simulink model "mcb_microchip_pmsm_parameter_est_SAME70"  (R2023b)
settings: Solver=FixedStepDiscrete  StartTime=0.0  StopTime=15  RelTol=1e-3  EnableMultiTasking=on
InitFcn:
  | mcb_microchip_pmsm_parameter_est_SAME70_data;
values from neighbouring files (symbols this model uses):
  Ts = T_pwm    (= 5e-05)    [mcb_microchip_pmsm_parameter_est_SAME70_data.m]
  Ts_motor = T_pwm/2    (= 2.5e-05)    [mcb_microchip_pmsm_parameter_est_SAME70_data.m]
undefined symbols (not defined in the file or in its folder): A24, AD10, AD7, ADC0, inverter, LQFP144, MaxPer, ms, ns, PA0, PA1, PA10, PA11, PA12, PA13, PA16, PA18, PA9, PB0, PD18, PD19, PD24, PD25, PD26, PI_params, Pin, pmsm, Resol, SAME70Q21B, target, Unsigned
libraries: simulink x18, MCHP_Blockset x13, mcbpmsmparamestlib x5, svdutilitieslib x4, mcbpositiondecoderlib x3, mcbplantlib x1, autolibpmsmexterior x1, mcbcontrolslib x1
(part 1 of 4)
settings Model: Creator=Lubin Kerhuel  LastModifiedBy=I69995
settings SolverCC: AlgebraicLoopSolver=TrustRegion
settings DataIOCC: SaveFormat=StructureWithTime  ReturnWorkspaceOutputs=off
settings OptimizationCC: DefaultParameterBehavior=Inlined  DefaultUnderspecifiedDataType=single  EnhancedBackFolding=on  PassReuseOutputArgsAs=Individual arguments  OptimizeBlockOrder=speed  DifferentSizesBufferReuse=on  OptimizationCustomize=off  EfficientTunableParamExpr=on
settings DebuggingCC: MultiTaskDSMMsg=none  ParameterPrecisionLossMsg=none  ParameterTunabilityLossMsg=error  FcnCallInpInsideContextMsg=warning  UnconnectedInputMsg=warning  UnconnectedOutputMsg=warning  UnconnectedLineMsg=warning  SFExecutionAtInitializationDiag=none  ArithmeticOperatorsInVariantConditions=warning
settings HardwareCC: ProdBitPerPointer=32  ProdBitPerSizeT=32  ProdBitPerPtrDiffT=32  ProdLargestAtomicInteger=Integer  ProdWordSize=32  ProdLongLongMode=on  ProdHWDeviceType=ARM Compatible->ARM Cortex
settings ModelReferenceCC: EnableRefExpFcnMdlSchedulingChecks=on  ModelReferenceNumInstancesAllowed=Single  PropagateSignalLabelsOutOfModel=off
settings SFSimCC: SimUseLocalCustomCode=off  MATLABDynamicMemAlloc=off  CustomCodeUndefinedFunction=UseInterfaceOnly
settings RTWCC: Description=Microchip Embedded Target Cortex M7 (real-time)  SystemTargetFile=MCHP_ARM7_stf.tlc  TemplateMakefile=MCHP_ARM7.tmf  GenerateReport=on  RTWUseLocalCustomCode=off  Toolchain=xc32 - v4.30 for Mirochip SAMx7 device  BuildConfiguration=Specify  IncludeHyperlinkInReport=on  LaunchReport=on  GenerateTraceInfo=on  GenerateTraceReport=on  GenerateTraceReportSl=on  GenerateTraceReportSf=on  GenerateTraceReportEml=on  DLArmComputeVersion=19.05
settings CodeAppCC: ForceParamTrailComments=on  IgnoreCustomStorageClasses=off  MaxIdLength=255  OperatorAnnotations=on  SimulinkDataObjDesc=on  SFDataObjDesc=on  InsertBlockDesc=on  InternalIdentifier=Classic
settings STFCustomTargetCC: TargetLangStandard=C89/C90 (ANSI)  MultiwordLength=256  IncludeMdlTerminateFcn=off  CombineOutputUpdateFcns=on  CombineSignalStateStructs=on  SuppressErrorStatus=on  ERTCustomFileBanners=on  SupportContinuousTime=off  RemoveResetFunc=on  MATLABClassNameForMDSCustomization=Simulink.SoftwareTarget.ERTCustomization  UseToolchainInfoCompliant=on  SystemTargetFile=MCHP_ARM7_stf.tlc
settings ERTTargetCC: ParMdlRefBuildCompliant=off  CompOptLevelCompliant=off  ConcurrentExecutionCompliant=off  IncludeMdlTerminateFcn=off  CombineSignalStateStructs=on  SuppressErrorStatus=on  SupportNonInlinedSFcns=on  ModelStepFunctionPrototypeControlCompliant=off  CPPClassGenCompliant=off  ExtModeStaticAllocSize=2000  InlinedParameterPlacement=NonHierarchical  ERTSrcFileBannerTemplate=MCHP_dsPIC_code_template.cgt  ERTHdrFileBannerTemplate=MCHP_dsPIC_code_template.cgt  ERTDataSrcFileTemplate=MCHP_dsPIC_code_template.cgt  ERTDataHdrFileTemplate=MCHP_dsPIC_code_template.cgt  ERTCustomFileTemplate=MCHP_main.tlc

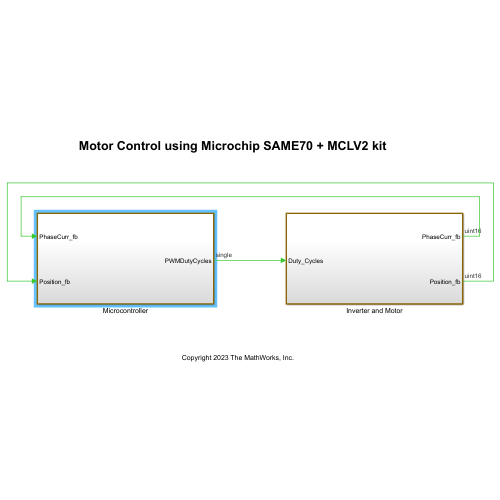
[thumbnail: Simulink's stored preview of the top-level diagram]
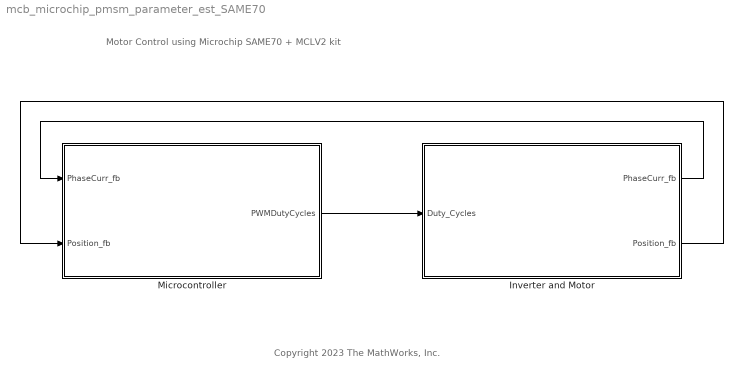
== system mcb_microchip_pmsm_parameter_est_SAME70 ==
  note: Copyright 2023 The MathWorks, Inc.
  note: Motor Control using Microchip SAME70 + MCLV2 kit
  Inverter and Motor : Subsystem
  Microcontroller : Subsystem
  wires:
  Microcontroller/1(PWMDutyCycles) -> Inverter and Motor/1(Duty_Cycles)
  Inverter and Motor/1(PhaseCurr_fb) -> Microcontroller/1(PhaseCurr_fb)
  Inverter and Motor/2(Position_fb) -> Microcontroller/2(Position_fb)

== system mcb_microchip_pmsm_parameter_est_SAME70/Inverter and Motor ==
  Duty_Cycles : Inport
  Inverter and Motor : Subsystem  Variant=on  VariantControlMode=sim codegen switching
  PhaseCurr_fb : Outport
  Position_fb : Outport  Port=2
  wires:
  Duty_Cycles/1 -> Inverter and Motor/1(Duty_Cycles)
  Inverter and Motor/1(PhaseCurr_fb) -> PhaseCurr_fb/1
  Inverter and Motor/2(Position_fb) -> Position_fb/1

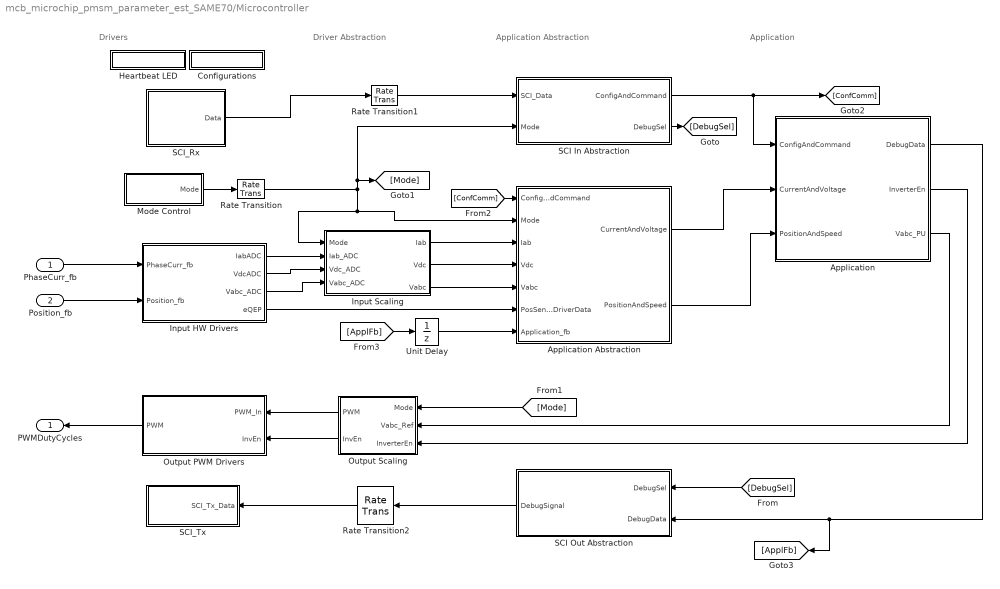
== system mcb_microchip_pmsm_parameter_est_SAME70/Microcontroller ==
  note: Drivers
  note: Driver Abstraction
  note: Application Abstraction
  note: Application
  PhaseCurr_fb : Inport
  Position_fb : Inport  Port=2
  Application : Subsystem
  Application Abstraction : Subsystem
  Configurations : Subsystem
  Heartbeat LED : Subsystem  Variant=on  VariantControlMode=sim codegen switching
  Input HW Drivers : Subsystem  Variant=on  VariantControlMode=sim codegen switching
  Input Scaling : Subsystem
  Mode Control : Subsystem  Variant=on
  Output PWM Drivers : Subsystem  Variant=on  VariantControlMode=sim codegen switching
  Output Scaling : Subsystem
  Rate Transition : RateTransition  Deterministic=off  OutPortSampleTime=Ts
  Rate Transition1 : RateTransition  Deterministic=off  OutPortSampleTime=Ts
  Rate Transition2 : RateTransition  Deterministic=off  OutPortSampleTime=Ts_SerialCom
  SCI In Abstraction : Subsystem
  SCI Out Abstraction : Subsystem
  SCI_Rx : Subsystem
  SCI_Tx : Subsystem  Variant=on  VariantControlMode=sim codegen switching
  Unit Delay : UnitDelay  SampleTime=-1  HasFrameUpgradeWarning=on
  PWMDutyCycles : Outport
  wires:
  SCI In Abstraction/1(ConfigAndCommand) -> Application/1(ConfigAndCommand), [ConfComm]
  Application Abstraction/1(CurrentAndVoltage) -> Application/2(CurrentAndVoltage)
  Application Abstraction/2(PositionAndSpeed) -> Application/3(PositionAndSpeed)
  Input Scaling/1(Iab) -> Application Abstraction/3(Iab)
  Input Scaling/2(Vdc) -> Application Abstraction/4(Vdc)
  Input Scaling/3(Vabc) -> Application Abstraction/5(Vabc)
  Application/1(DebugData) -> SCI Out Abstraction/2(DebugData), [ApplFb]
  Unit Delay/1 -> Application Abstraction/7(Application_fb)
  Rate Transition/1 -> Application Abstraction/2(Mode), Input Scaling/1(Mode), [Mode], SCI In Abstraction/2(Mode)
  Rate Transition1/1 -> SCI In Abstraction/1(SCI_Data)
  SCI_Rx/1(Data) -> Rate Transition1/1
  Position_fb/1 -> Input HW Drivers/2(Position_fb)
  PhaseCurr_fb/1 -> Input HW Drivers/1(PhaseCurr_fb)
  Input HW Drivers/1(IabADC) -> Input Scaling/2(Iab_ADC)
  Input HW Drivers/2(VdcADC) -> Input Scaling/3(Vdc_ADC)
  Input HW Drivers/3(Vabc_ADC) -> Input Scaling/4(Vabc_ADC)
  Input HW Drivers/4(eQEP) -> Application Abstraction/6(PosSenseDriverData)
  Application/3(Vabc_PU) -> Output Scaling/2(Vabc_Ref)
  Application/2(InverterEn) -> Output Scaling/3(InverterEn)
  SCI In Abstraction/2(DebugSel) -> [DebugSel]
  [DebugSel] -> SCI Out Abstraction/1(DebugSel)
  [Mode] -> Output Scaling/1(Mode)
  [ConfComm] -> Application Abstraction/1(ConfigAndCommand)
  [ApplFb] -> Unit Delay/1
  Output PWM Drivers/1(PWM) -> PWMDutyCycles/1
  Output Scaling/1(PWM) -> Output PWM Drivers/1(PWM_In)
  Output Scaling/2(InvEn) -> Output PWM Drivers/2(InvEn)
  SCI Out Abstraction/1(DebugSignal) -> Rate Transition2/1
  Mode Control/1(Mode) -> Rate Transition/1
  Rate Transition2/1 -> SCI_Tx/1(SCI_Tx_Data)

== system mcb_microchip_pmsm_parameter_est_SAME70/Inverter and Motor/Inverter and Motor ==
  Duty_Cycles : Inport
  Codegen : Subsystem  VariantControl=(codegen)
  Sim : Subsystem  VariantControl=(sim)
  PhaseCurr_fb : Outport
  Position_fb : Outport  Port=2

== system mcb_microchip_pmsm_parameter_est_SAME70/Microcontroller/Application ==
  ConfigAndCommand : Inport
  CurrentAndVoltage : Inport  Port=2
  PositionAndSpeed : Inport  Port=3
  Bus Creator : BusCreator  Inputs=5
  Bus Selector2 : BusSelector  OutputSignals=Enable,TestMethod,TestSelect,Config
  Bus Selector4 : BusSelector  OutputSignals=Theta,Speed,EnClosedLoop
  Bus Selector5 : BusSelector  OutputSignals=Iabc,Vdc
  Param Est : Subsystem
  DebugData : Outport
  InverterEn : Outport  Port=2
  Vabc_PU : Outport  Port=3
  wires:
  ConfigAndCommand/1 -> Bus Selector2/1
  PositionAndSpeed/1 -> Bus Selector4/1
  CurrentAndVoltage/1 -> Bus Selector5/1
  Bus Creator/1 -> Param Est/1(HWInputs)
  Bus Selector5/2 -> Bus Creator/2  "<Vdc>"
  Bus Selector5/1 -> Bus Creator/1  "<Iabc>"
  Bus Selector4/1 -> Bus Creator/3  "<Theta>"
  Bus Selector4/2 -> Bus Creator/4  "<Speed>"
  Bus Selector4/3 -> Bus Creator/5  "<EnClosedLoop>"
  Bus Selector2/4 -> Param Est/5(Config)  "<Config>"
  Bus Selector2/3 -> Param Est/4(TestSelect)  "<TestSelect>"
  Bus Selector2/2 -> Param Est/3(TestMethod)  "<TestMethod>"
  Bus Selector2/1 -> Param Est/2(Enable)  "<Enable>"
  Param Est/2(InverterEn) -> InverterEn/1
  Param Est/1(Vabc) -> Vabc_PU/1
  Param Est/3(DebugData) -> DebugData/1

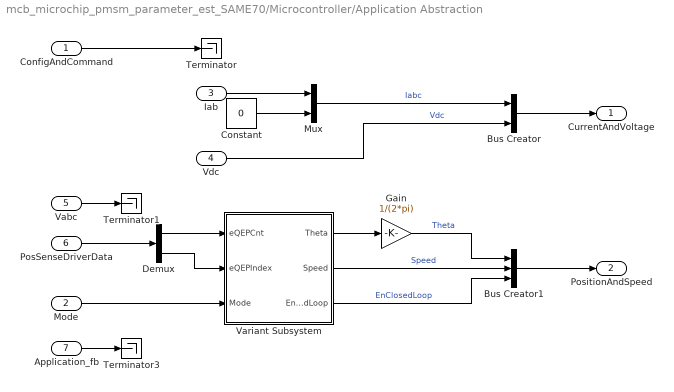
== system mcb_microchip_pmsm_parameter_est_SAME70/Microcontroller/Application Abstraction ==
  ConfigAndCommand : Inport
  Mode : Inport  Port=2
  Iab : Inport  Port=3
  Vdc : Inport  Port=4
  Vabc : Inport  Port=5
  PosSenseDriverData : Inport  Port=6
  Application_fb : Inport  Port=7
  Bus Creator : BusCreator  Inputs=2
  Bus Creator1 : BusCreator  Inputs=3
  Constant : Constant  Value=0  OutDataTypeStr=single
  Demux : Demux  Outputs=2
  Gain : Gain  Gain=1/(2*pi)  RndMeth=Simplest  OutDataTypeStr=Inherit: Same as input
  Mux : Mux  Inputs=2
  Terminator : Terminator
  Terminator1 : Terminator
  Terminator3 : Terminator
  Variant Subsystem : Subsystem  Variant=on
  CurrentAndVoltage : Outport
  PositionAndSpeed : Outport  Port=2
  wires:
  ConfigAndCommand/1 -> Terminator/1
  Iab/1 -> Mux/1
  Mux/1 -> Bus Creator/1  "Iabc"
  Bus Creator/1 -> CurrentAndVoltage/1
  Bus Creator1/1 -> PositionAndSpeed/1
  Variant Subsystem/2(Speed) -> Bus Creator1/2  "Speed"
  Variant Subsystem/1(Theta) -> Gain/1
  Variant Subsystem/3(EnClosedLoop) -> Bus Creator1/3  "EnClosedLoop"
  Mode/1 -> Variant Subsystem/3(Mode)
  PosSenseDriverData/1 -> Demux/1
  Demux/1 -> Variant Subsystem/1(eQEPCnt)
  Demux/2 -> Variant Subsystem/2(eQEPIndex)
  Vabc/1 -> Terminator1/1
  Vdc/1 -> Bus Creator/2  "Vdc"
  Application_fb/1 -> Terminator3/1
  Constant/1 -> Mux/2
  Gain/1 -> Bus Creator1/1  "Theta"
